simulink model "DC_DC_converter_closed_loop"  (R2019a)
settings: Solver=ode23tb  StartTime=0.0  StopTime=0.28  MaxStep=1e-7  RelTol=1e-7
values from neighbouring files (symbols this model uses):
  C = 33e-6    (= 3.3e-05)    [parameters_for_boost_converter_closed_loop.m]    (also in parameters_for_buck_converter_closed_loop.m)
  D = 1-((Vg+sqrt(Vg^2-4*V^2*((RL+Rdson)/R)))/(2*V))    [parameters_for_boost_converter_closed_loop.m]    (also in parameters_for_buck_converter_closed_loop.m = 0.425529411765)
  fsw = 100e3    (= 100000)    [parameters_for_boost_converter_closed_loop.m]    (also in parameters_for_buck_converter_closed_loop.m)
  H = 0.0075    [parameters_for_boost_converter_closed_loop.m]    (also in parameters_for_buck_converter_closed_loop.m)
  I = V/(R*(1-D))    [parameters_for_boost_converter_closed_loop.m]    (also in parameters_for_buck_converter_closed_loop.m = 11.7647058824)
  Kic_boost = 13590    [parameters_for_boost_converter_closed_loop.m]
  Kic_buck = 13529    [parameters_for_buck_converter_closed_loop.m]
  Kiv_boost = 25396    [parameters_for_boost_converter_closed_loop.m]
  Kiv_buck = 25428    [parameters_for_buck_converter_closed_loop.m]
  Kpc_boost = 0.618    [parameters_for_boost_converter_closed_loop.m]
  Kpc_buck = 0.6    [parameters_for_buck_converter_closed_loop.m]
  Kpv_boost = 15.62    [parameters_for_boost_converter_closed_loop.m]
  Kpv_buck = 6.53    [parameters_for_buck_converter_closed_loop.m]
  L = 250e-6    (= 0.00025)    [parameters_for_boost_converter_closed_loop.m]    (also in parameters_for_buck_converter_closed_loop.m)
  R = V/Iload    (= 80)    [parameters_for_boost_converter_closed_loop.m]    (also in parameters_for_buck_converter_closed_loop.m = 14.45)
  Resr = 6e-3    (= 0.006)    [parameters_for_boost_converter_closed_loop.m]    (also in parameters_for_buck_converter_closed_loop.m)
  Rf = 0.25    [parameters_for_boost_converter_closed_loop.m]    (also in parameters_for_buck_converter_closed_loop.m)
  RL = 10e-3    (= 0.01)    [parameters_for_boost_converter_closed_loop.m]    (also in parameters_for_buck_converter_closed_loop.m)
  Tsamp_dc = Tsw/2    (= 5e-06)    [parameters_for_boost_converter_closed_loop.m]    (also in parameters_for_buck_converter_closed_loop.m)
  V = 400    [parameters_for_boost_converter_closed_loop.m]    (also in parameters_for_buck_converter_closed_loop.m = 170)
  Vg = 170    [parameters_for_boost_converter_closed_loop.m]    (also in parameters_for_buck_converter_closed_loop.m = 400)
  VM = 4    [parameters_for_boost_converter_closed_loop.m]    (also in parameters_for_buck_converter_closed_loop.m)
  Vref = H*V    (= 3)    [parameters_for_boost_converter_closed_loop.m]    (also in parameters_for_buck_converter_closed_loop.m = 1.275)
libraries: powerlib x40, simulink x5
settings Model: Creator=Görkem  LastModifiedBy=gsahi
settings SolverCC: ZeroCrossAlgorithm=Adaptive
settings DebuggingCC: IgnoredZcDiagnostic=none

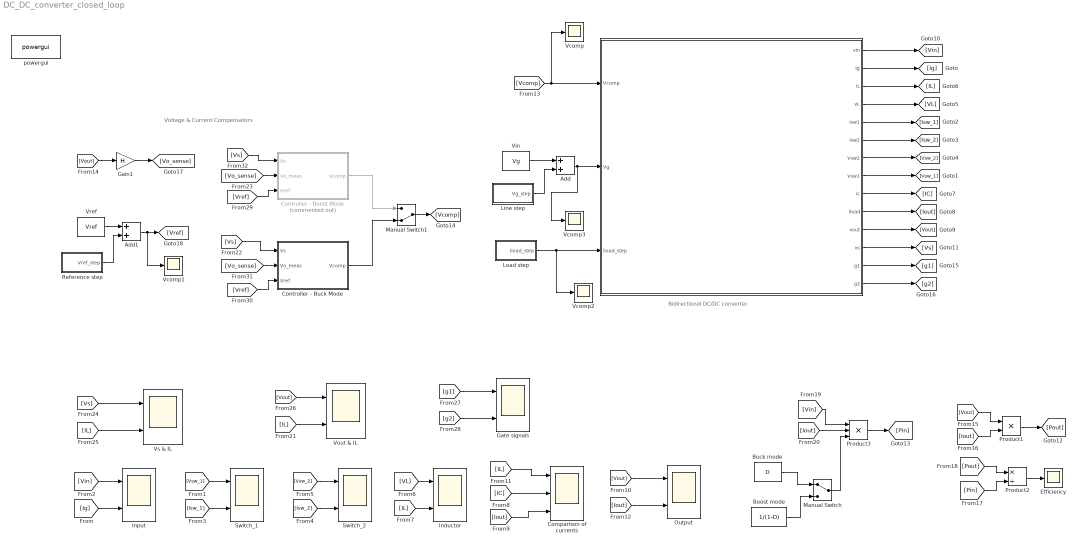
== system DC_DC_converter_closed_loop ==
  note: Voltage & Current Compensators
  note: Bidirectional DC/DC converter
  "   " : Subsystem
  Add : Sum
  Add1 : Sum
  Boost mode : Constant  Value=1/(1-D)
  Buck mode : Constant  Value=D
  Comparison of currents : Scope  NumInputPorts=3
  Controller - Boost Mode : Subsystem  Commented=on
  Controller - Buck Mode : Subsystem
  Efficiency : Scope
  Gain1 : Gain  Gain=H
  Gate signals : Scope  NumInputPorts=2
  Inductor : Scope  NumInputPorts=2
  Input : Scope  NumInputPorts=2
  Line step : Subsystem
  Load step : Subsystem
  Manual Switch : ManualSwitch
  Manual Switch1 : ManualSwitch  CurrentSetting=0
  "Output " : Scope  NumInputPorts=2
  Product1 : Product
  Product2 : Product  Inputs=*/
  Product3 : Product  Inputs=3
  Reference step : Subsystem
  Switch_1 : Scope  NumInputPorts=2
  Switch_2 : Scope  NumInputPorts=2
  Vcomp{,1..3} (4 alike) : Scope
  Vin : Constant  Value=Vg
  Vout & IL : Scope  NumInputPorts=2
  Vref : Constant  Value=Vref
  Vs & IL : Scope  NumInputPorts=2
  powergui : powerlib/powergui  Priority=1  SimulationMode=Continuous  SampleTime=5e-6  frequency=60  Iterations=50  frequencyindice=0  Pbase=100e6  ErrMax=1e-4  UnitsV=kV  UnitsW=MW  buscounter=0  FunctionMessages=off  echomessages=off  EnableUseOfTLC=off  CurrentSourceSwitches=off  DisableSnubberDevices=off  DisableRonSwitches=off  DisableVfSwitches=off  DisplayEquations=off  AutomaticDiscreteSolvers=off  SolverType=Tustin/Backward Euler (TBE)  Interpol=off  ExternalGateDelay=off  methode=off  Ts=100  x0status=blocks  SPID=on  SwTol=0  HookPort=off  NonlinearTolerance=0  nMaxIteration=15  ContinueOnMaxIteration=off  RestoreLinks=warning  ResistiveCurrentMeasurement=off  Frange=[0:2:500]  Ylog=off  Xlog=on  ShowGrid=off  save=off  variable=ZData  structure=0  ZoomFFT=off  StartTime=0.0  cycles=1  DisplayStyle=1  fundamental=60  FreqAxis=off  MaxFrequency=1000  frequencyindicesteady=1  RmsSteady=1  display=off
      settings: SourceProductName=Simscape Electrical
  wires:
  [Vin] -> Product3/1
  [Iout] -> Product3/2
  "   "/4(vL) -> [VL]
  "   "/6(isw2) -> [Isw_2]
  Product1/1 -> [Pout]
  "   "/9(ic) -> [IC]
  "   "/2(Ig) -> [Ig]
  "   "/11(vout) -> [Vout]
  Product3/1 -> [Pin]
  "   "/5(isw1) -> [Isw_1]
  [Vin] -> Input/1
  "   "/8(Vsw1) -> [Vsw_1]
  "   "/7(Vsw2) -> [Vsw_2]
  "   "/10(iload) -> [Iout]
  "   "/3(iL) -> [IL]
  [Iout] -> Comparison of currents/3
  [Pin] -> Product2/2
  [IL] -> Vout & IL/2
  [Pout] -> Product2/1
  "   "/1(vin) -> [Vin]
  Product2/1 -> Efficiency/1
  [Vout] -> Vout & IL/1
  [Isw_2] -> Switch_2/2
  [Iout] -> Product1/2
  [Vout] -> "Output "/1
  [IL] -> Inductor/2
  [VL] -> Inductor/1
  [Iout] -> "Output "/2
  [IC] -> Comparison of currents/2
  [Isw_1] -> Switch_1/2
  [Ig] -> Input/2
  [IL] -> Comparison of currents/1
  [Vsw_2] -> Switch_2/1
  [Vsw_1] -> Switch_1/1
  [Vout] -> Product1/1
  Buck mode/1 -> Manual Switch/1
  Boost mode/1 -> Manual Switch/2
  Manual Switch/1 -> Product3/3
  "   "/12(vs) -> [Vs]
  [Vout] -> Gain1/1
  [Vs] -> Vs & IL/1
  [IL] -> Vs & IL/2
  "   "/13(g1) -> [g1]
  "   "/14(g2) -> [g2]
  [g2] -> Gate signals/2
  [g1] -> Gate signals/1
  [Vcomp] -> Vcomp/1, "   "/1(Vcomp)
  Controller - Boost Mode/1("Vcomp ") -> Manual Switch1/1
  Controller - Buck Mode/1("Vcomp ") -> Manual Switch1/2
  Manual Switch1/1 -> [Vcomp]
  Gain1/1 -> [Vo_sense]
  [Vs] -> Controller - Buck Mode/1(Vs)
  [Vo_sense] -> Controller - Boost Mode/2(Vo_meas)
  [Vref] -> Controller - Boost Mode/3(Vref)
  [Vref] -> Controller - Buck Mode/3(Vref)
  [Vo_sense] -> Controller - Buck Mode/2(Vo_meas)
  [Vs] -> Controller - Boost Mode/1(Vs)
  Vin/1 -> Add/1
  Add/1 -> Vcomp3/1, "   "/2(Vg)
  Line step/1(Vg_step) -> Add/2
  Vref/1 -> Add1/1
  Reference step/1(Vref_step) -> Add1/2
  Add1/1 -> Vcomp1/1, [Vref]
  Load step/1(Iload_step) -> Vcomp2/1, "   "/3(iload_step)

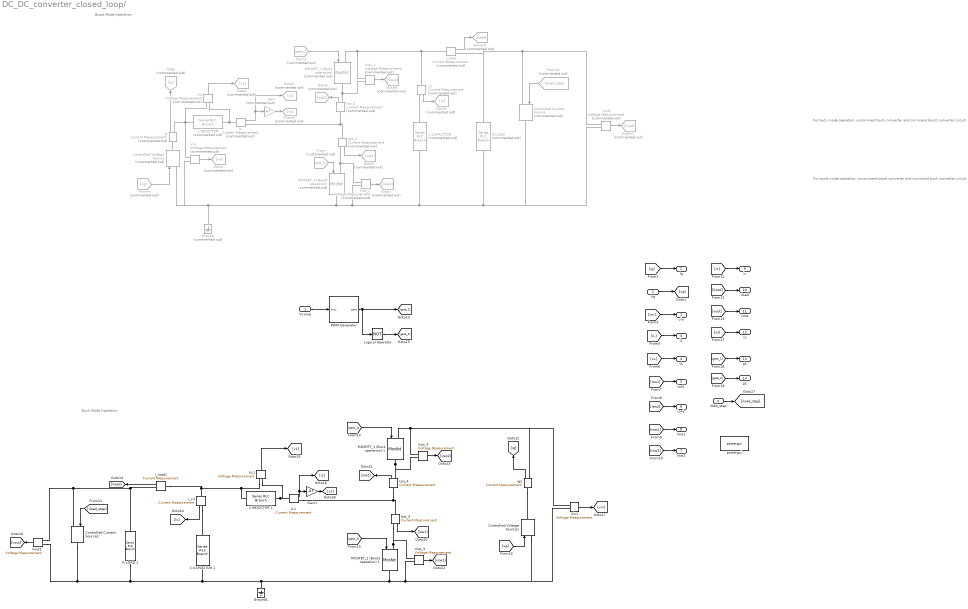
== system DC_DC_converter_closed_loop/    ==
  note: For buck mode operation, uncomment buck converter and command boost converter circuit
  note: Buck Mode Operation
  note: Boost Mode Operation
  note: For boost mode operation, uncomment boost converter and command buck converter circuit
  Vcomp : Inport
  Vg : Inport  Port=2
  iload_step : Inport  Port=3
  "C:CAPACITOR " : powerlib/Elements/Series RLC Branch  Commented=on  LConnTagsString=__new0  RConnTagsString=__new0  BranchType=RC  Resistance=Resr  Inductance=1e-3  SetiL0=off  InitialCurrent=0  Capacitance=C  Setx0=off  InitialVoltage=0  Measurements=None
      settings: SourceProductName=Simscape Electrical
  C:CAPACITOR 1 : powerlib/Elements/Series RLC Branch  LConnTagsString=__new0  RConnTagsString=__new0  BranchType=RC  Resistance=Resr  Inductance=1e-3  SetiL0=off  InitialCurrent=0  Capacitance=C  Setx0=off  InitialVoltage=0  Measurements=None
      settings: SourceProductName=Simscape Electrical
  Controlled Current Source : powerlib/Electrical Sources/Controlled Current Source  Commented=on  Initialize=on  Source_Type=AC  Amplitude=0  Phase=0  Frequency=0  Measurements=None
      settings: SourceProductName=Simscape Electrical
  Controlled Current Source1 : powerlib/Electrical Sources/Controlled Current Source  Initialize=on  Source_Type=AC  Amplitude=0  Phase=0  Frequency=0  Measurements=None
      settings: SourceProductName=Simscape Electrical
  Controlled Voltage Source : powerlib/Electrical Sources/Controlled Voltage Source  Commented=on  Initialize=on  Source_Type=DC  Amplitude=0  Phase=0  Frequency=0  Measurements=None
      settings: SourceProductName=Simscape Electrical
  Controlled Voltage Source1 : powerlib/Electrical Sources/Controlled Voltage Source  Initialize=on  Source_Type=DC  Amplitude=0  Phase=0  Frequency=0  Measurements=None
      settings: SourceProductName=Simscape Electrical
  From : From  Commented=on  GotoTag=gate_1
  From1 : From  Commented=on  GotoTag=gate_2
  From20 : From  Commented=on  GotoTag=iload_step
  From4 : From  Commented=on  GotoTag=vg
  Gain : Gain  Commented=on  Gain=Rf
  Gain1 : Gain  Gain=-Rf
  Goto : Goto  Commented=on  GotoTag=ig
  Goto10 : Goto  Commented=on  GotoTag=iload
  Goto11 : Goto  Commented=on  GotoTag=vout
  Goto2 : Goto  Commented=on  GotoTag=vin
  Goto25 : Goto  Commented=on  GotoTag=vs
  Goto3 : Goto  Commented=on  GotoTag=iL
  Goto4 : Goto  Commented=on  GotoTag=vL
  Goto5 : Goto  Commented=on  GotoTag=isw1
  Goto6 : Goto  Commented=on  GotoTag=isw2
  Goto7 : Goto  Commented=on  GotoTag=vsw1
  Goto8 : Goto  Commented=on  GotoTag=vsw2
  Goto9 : Goto  Commented=on  GotoTag=ic
  Ground : powerlib/Elements/Ground  Commented=on  LConnTagsString=a
      settings: SourceProductName=Simscape Electrical
  Ground1 : powerlib/Elements/Ground  LConnTagsString=a
      settings: SourceProductName=Simscape Electrical
  IL : powerlib/Measurements/Current Measurement  Commented=on  PhasorSimulation=off  OutputType=Complex  PSBequivalent=0
      settings: SourceProductName=Simscape Electrical
  IL1 : powerlib/Measurements/Current Measurement  PhasorSimulation=off  OutputType=Complex  PSBequivalent=0
      settings: SourceProductName=Simscape Electrical
  Isw_1 : powerlib/Measurements/Current Measurement  Commented=on  PhasorSimulation=off  OutputType=Complex  PSBequivalent=0
      settings: SourceProductName=Simscape Electrical
  Isw_2 : powerlib/Measurements/Current Measurement  Commented=on  PhasorSimulation=off  OutputType=Complex  PSBequivalent=0
      settings: SourceProductName=Simscape Electrical
  Isw_3 : powerlib/Measurements/Current Measurement  PhasorSimulation=off  OutputType=Complex  PSBequivalent=0
      settings: SourceProductName=Simscape Electrical
  Isw_4 : powerlib/Measurements/Current Measurement  PhasorSimulation=off  OutputType=Complex  PSBequivalent=0
      settings: SourceProductName=Simscape Electrical
  "L:INDUCTOR " : powerlib/Elements/Series RLC Branch  Commented=on  LConnTagsString=__new0  RConnTagsString=__new0  BranchType=RL  Resistance=RL  Inductance=L  SetiL0=off  InitialCurrent=0  Capacitance=1e-6  Setx0=off  InitialVoltage=0  Measurements=None
      settings: SourceProductName=Simscape Electrical
  L:INDUCTOR 1 : powerlib/Elements/Series RLC Branch  LConnTagsString=__new0  RConnTagsString=__new0  BranchType=RL  Resistance=RL  Inductance=L  SetiL0=off  InitialCurrent=0  Capacitance=1e-6  Setx0=off  InitialVoltage=0  Measurements=None
      settings: SourceProductName=Simscape Electrical
  Logical Operator : Logic  Operator=NOT  AllPortsSameDT=off  OutDataTypeStr=boolean
  "MOSFET_1 (Buck operation) " : powerlib/Power Electronics/Mosfet  Commented=on  Ron=Rdson  Lon=0  Rd=0  Vfd=Vf  IC=0  Rs=1e5  Cs=inf  Measurements=off
      settings: SourceProductName=Simscape Electrical
  MOSFET_1 (Buck operation) 1 : powerlib/Power Electronics/Mosfet  Ron=Rdson  Lon=0  Rd=0  Vfd=Vf  IC=0  Rs=1e5  Cs=inf  Measurements=off
      settings: SourceProductName=Simscape Electrical
  "MOSFET_2 (Boost operation) " : powerlib/Power Electronics/Mosfet  Commented=on  Ron=Rdson  Lon=0  Rd=0  Vfd=Vf  IC=0  Rs=1e5  Cs=inf  Measurements=off
      settings: SourceProductName=Simscape Electrical
  MOSFET_2 (Boost operation) 1 : powerlib/Power Electronics/Mosfet  Ron=Rdson  Lon=0  Rd=0  Vfd=Vf  IC=0  Rs=1e5  Cs=inf  Measurements=off
      settings: SourceProductName=Simscape Electrical
  PWM Generator : Subsystem
  "R:LOAD " : powerlib/Elements/Series RLC Branch  Commented=on  LConnTagsString=__new0  RConnTagsString=__new0  BranchType=R  Resistance=R  Inductance=1e-3  SetiL0=off  InitialCurrent=0  Capacitance=47e-6  Setx0=off  InitialVoltage=0  Measurements=None
      settings: SourceProductName=Simscape Electrical
  R:LOAD 1 : powerlib/Elements/Series RLC Branch  LConnTagsString=__new0  RConnTagsString=__new0  BranchType=R  Resistance=R  Inductance=1e-3  SetiL0=off  InitialCurrent=0  Capacitance=47e-6  Setx0=off  InitialVoltage=0  Measurements=None
      settings: SourceProductName=Simscape Electrical
  VL : powerlib/Measurements/Voltage Measurement  Commented=on  PhasorSimulation=off  OutputType=Complex  PSBequivalent=0
      settings: SourceProductName=Simscape Electrical
  VL1 : powerlib/Measurements/Voltage Measurement  PhasorSimulation=off  OutputType=Complex  PSBequivalent=0
      settings: SourceProductName=Simscape Electrical
  Vin : powerlib/Measurements/Voltage Measurement  Commented=on  PhasorSimulation=off  OutputType=Complex  PSBequivalent=0
      settings: SourceProductName=Simscape Electrical
  Vin1 : powerlib/Measurements/Voltage Measurement  PhasorSimulation=off  OutputType=Complex  PSBequivalent=0
      settings: SourceProductName=Simscape Electrical
  Vout : powerlib/Measurements/Voltage Measurement  Commented=on  PhasorSimulation=off  OutputType=Complex  PSBequivalent=0
      settings: SourceProductName=Simscape Electrical
  Vout1 : powerlib/Measurements/Voltage Measurement  PhasorSimulation=off  OutputType=Complex  PSBequivalent=0
      settings: SourceProductName=Simscape Electrical
  Vsw_1 : powerlib/Measurements/Voltage Measurement  Commented=on  PhasorSimulation=off  OutputType=Complex  PSBequivalent=0
      settings: SourceProductName=Simscape Electrical
  Vsw_2 : powerlib/Measurements/Voltage Measurement  Commented=on  PhasorSimulation=off  OutputType=Complex  PSBequivalent=0
      settings: SourceProductName=Simscape Electrical
  Vsw_3 : powerlib/Measurements/Voltage Measurement  PhasorSimulation=off  OutputType=Complex  PSBequivalent=0
      settings: SourceProductName=Simscape Electrical
  Vsw_4 : powerlib/Measurements/Voltage Measurement  PhasorSimulation=off  OutputType=Complex  PSBequivalent=0
      settings: SourceProductName=Simscape Electrical
  i_c : powerlib/Measurements/Current Measurement  Commented=on  PhasorSimulation=off  OutputType=Complex  PSBequivalent=0
      settings: SourceProductName=Simscape Electrical
  i_c1 : powerlib/Measurements/Current Measurement  PhasorSimulation=off  OutputType=Complex  PSBequivalent=0
      settings: SourceProductName=Simscape Electrical
  i_load : powerlib/Measurements/Current Measurement  Commented=on  PhasorSimulation=off  OutputType=Complex  PSBequivalent=0
      settings: SourceProductName=Simscape Electrical
  i_load1 : powerlib/Measurements/Current Measurement  PhasorSimulation=off  OutputType=Complex  PSBequivalent=0
      settings: SourceProductName=Simscape Electrical
  ig : powerlib/Measurements/Current Measurement  Commented=on  PhasorSimulation=off  OutputType=Complex  PSBequivalent=0
      settings: SourceProductName=Simscape Electrical
  ig1 : powerlib/Measurements/Current Measurement  PhasorSimulation=off  OutputType=Complex  PSBequivalent=0
      settings: SourceProductName=Simscape Electrical
  powergui : powerlib/powergui  Priority=1  SimulationMode=Continuous  SampleTime=50e-6  frequency=60  Iterations=50  frequencyindice=0  Pbase=100e6  ErrMax=1e-4  UnitsV=kV  UnitsW=MW  buscounter=0  FunctionMessages=off  echomessages=off  EnableUseOfTLC=off  CurrentSourceSwitches=off  DisableSnubberDevices=off  DisableRonSwitches=off  DisableVfSwitches=off  DisplayEquations=off  AutomaticDiscreteSolvers=off  SolverType=Tustin/Backward Euler (TBE)  Interpol=off  ExternalGateDelay=off  methode=off  Ts=100  x0status=blocks  SPID=on  SwTol=0  HookPort=off  NonlinearTolerance=0  nMaxIteration=15  ContinueOnMaxIteration=off  RestoreLinks=warning  ResistiveCurrentMeasurement=off  Frange=[0:2:500]  Ylog=off  Xlog=on  ShowGrid=off  save=off  variable=ZData  structure=0  ZoomFFT=off  StartTime=0.0  cycles=1  DisplayStyle=1  fundamental=60  FreqAxis=off  MaxFrequency=1000  frequencyindicesteady=1  RmsSteady=1  display=off
      settings: SourceProductName=Simscape Electrical
  vin : Outport
  Ig : Outport  Port=2
  iL : Outport  Port=3
  vL : Outport  Port=4
  isw1 : Outport  Port=5
  isw2 : Outport  Port=6
  Vsw2 : Outport  Port=7
  Vsw1 : Outport  Port=8
  ic : Outport  Port=9
  iload : Outport  Port=10
  vout : Outport  Port=11
  vs : Outport  Port=12
  g1 : Outport  Port=13
  g2 : Outport  Port=14
  wires:
  PWM Generator/1(gate) -> Logical Operator/1, [gate_1]
  Logical Operator/1 -> [gate_2]
  Vcomp/1 -> PWM Generator/1(duty)
  From/1 -> "MOSFET_2 (Boost operation) "/1
  From1/1 -> "MOSFET_1 (Buck operation) "/1
  Vout/1 -> Goto11/1
  IL/1 -> Gain/1, Goto3/1
  VL/1 -> Goto4/1
  ig/1 -> Goto/1
  Isw_1/1 -> Goto5/1
  Isw_2/1 -> Goto6/1
  Vsw_1/1 -> Goto7/1
  Vsw_2/1 -> Goto8/1
  i_c/1 -> Goto9/1
  [ig] -> Ig/1
  Vg/1 -> [vg]
  From4/1 -> Controlled Voltage Source/1
  Vin/1 -> Goto2/1
  [vin] -> vin/1
  [iL] -> iL/1
  [vL] -> vL/1
  [isw1] -> isw1/1
  [isw2] -> isw2/1
  [vsw1] -> Vsw1/1
  [vsw2] -> Vsw2/1
  [ic] -> ic/1
  [iload] -> iload/1
  [vout] -> vout/1
  [gate_1] -> MOSFET_1 (Buck operation) 1/1
  Vsw_4/1 -> [vsw2]
  [gate_2] -> MOSFET_2 (Boost operation) 1/1
  VL1/1 -> [vL]
  Vsw_3/1 -> [vsw1]
  Isw_3/1 -> [isw1]
  IL1/1 -> [iL], Gain1/1
  Isw_4/1 -> [isw2]
  [vg] -> Controlled Voltage Source1/1
  ig1/1 -> [ig]
  Vin1/1 -> [vin]
  Vout1/1 -> [vout]
  i_c1/1 -> [ic]
  [vs] -> vs/1
  [gate_2] -> g2/1
  [gate_1] -> g1/1
  Gain/1 -> Goto25/1
  Gain1/1 -> [vs]
  From20/1 -> Controlled Current Source/1
  iload_step/1 -> [iload_step]
  i_load/1 -> Goto10/1
  [iload_step] -> Controlled Current Source1/1
  i_load1/1 -> [iload]
  connections:
  Vout/LConn1 -- i_load/RConn1 -- "R:LOAD "/LConn1 -- Controlled Current Source/LConn1
  "C:CAPACITOR "/RConn1 -- Controlled Current Source/RConn1 -- Vout/LConn2 -- "R:LOAD "/RConn1 -- Vsw_1/LConn2 -- Vin/LConn2 -- Controlled Voltage Source/LConn1 -- Ground/LConn1 -- "MOSFET_2 (Boost operation) "/RConn1
  Isw_1/LConn1 -- IL/RConn1 -- Isw_2/LConn1
  VL/LConn1 -- Vin/LConn1 -- "L:INDUCTOR "/LConn1 -- ig/RConn1
  IL/LConn1 -- VL/LConn2 -- "L:INDUCTOR "/RConn1
  ig/LConn1 -- Controlled Voltage Source/RConn1
  Isw_1/RConn1 -- Vsw_1/LConn1 -- "MOSFET_2 (Boost operation) "/LConn1
  Isw_2/RConn1 -- Vsw_2/LConn1 -- "MOSFET_1 (Buck operation) "/RConn1
  i_c/RConn1 -- "C:CAPACITOR "/LConn1
  MOSFET_1 (Buck operation) 1/RConn1 -- Isw_4/RConn1 -- Vsw_4/LConn1
  MOSFET_2 (Boost operation) 1/LConn1 -- Isw_3/RConn1 -- Vsw_3/LConn1
  Vout1/LConn2 -- Ground1/LConn1 -- Vin1/LConn2 -- Controlled Voltage Source1/LConn1 -- Vsw_3/LConn2 -- MOSFET_2 (Boost operation) 1/RConn1 -- C:CAPACITOR 1/RConn1 -- R:LOAD 1/RConn1 -- Controlled Current Source1/RConn1
  Isw_4/LConn1 -- Isw_3/LConn1 -- IL1/RConn1
  L:INDUCTOR 1/RConn1 -- IL1/LConn1 -- VL1/LConn2
  Vout1/LConn1 -- Controlled Current Source1/LConn1 -- i_load1/RConn1 -- R:LOAD 1/LConn1
  i_c1/RConn1 -- C:CAPACITOR 1/LConn1
  Vsw_4/LConn2 -- Vin1/LConn1 -- ig1/RConn1 -- MOSFET_1 (Buck operation) 1/LConn1
  ig1/LConn1 -- Controlled Voltage Source1/RConn1
  i_c/LConn1 -- i_load/LConn1 -- Vsw_2/LConn2 -- "MOSFET_1 (Buck operation) "/LConn1
  L:INDUCTOR 1/LConn1 -- i_load1/LConn1 -- i_c1/LConn1 -- VL1/LConn1

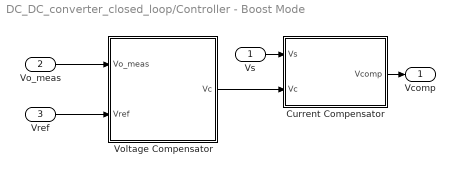
== system DC_DC_converter_closed_loop/Controller - Boost Mode ==
  Vs : Inport
  Vo_meas : Inport  Port=2
  Vref : Inport  Port=3
  Current Compensator : Subsystem
  "Voltage Compensator " : Subsystem
  "Vcomp " : Outport
  wires:
  Vs/1 -> Current Compensator/1(Vs)
  "Voltage Compensator "/1(Vc) -> Current Compensator/2(Vc)
  Vref/1 -> "Voltage Compensator "/2(Vref)
  Current Compensator/1(Vcomp) -> "Vcomp "/1
  Vo_meas/1 -> "Voltage Compensator "/1("Vo_meas ")

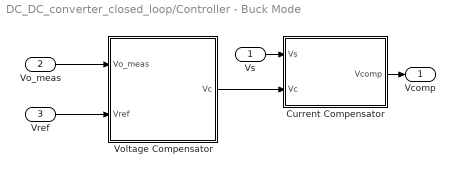
== system DC_DC_converter_closed_loop/Controller - Buck Mode ==
  Vs : Inport
  Vo_meas : Inport  Port=2
  Vref : Inport  Port=3
  Current Compensator : Subsystem
  "Voltage Compensator " : Subsystem
  "Vcomp " : Outport
  wires:
  Vs/1 -> Current Compensator/1(Vs)
  "Voltage Compensator "/1(Vc) -> Current Compensator/2(Vc)
  Vref/1 -> "Voltage Compensator "/2(Vref)
  Current Compensator/1(Vcomp) -> "Vcomp "/1
  Vo_meas/1 -> "Voltage Compensator "/1("Vo_meas ")

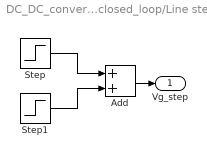
== system DC_DC_converter_closed_loop/Line step ==
  Add : Sum
  Step : Step  Time=0.12  After=10  SampleTime=0
  Step1 : Step  Time=0.16  After=-10  SampleTime=0
  Vg_step : Outport
  wires:
  Add/1 -> Vg_step/1
  Step/1 -> Add/1
  Step1/1 -> Add/2

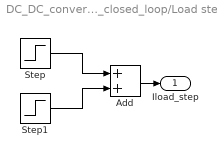
== system DC_DC_converter_closed_loop/Load step ==
  Add : Sum
  Step : Step  Time=0.20  After=V/R  SampleTime=0
  Step1 : Step  Time=0.24  After=-V/R  SampleTime=0
  Iload_step : Outport
  wires:
  Add/1 -> Iload_step/1
  Step/1 -> Add/1
  Step1/1 -> Add/2

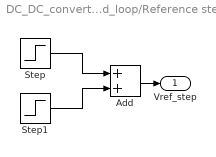
== system DC_DC_converter_closed_loop/Reference step ==
  Add : Sum
  Step : Step  Time=0.04  After=H*V*0.5  SampleTime=0
  Step1 : Step  Time=0.08  After=-H*V*0.5  SampleTime=0
  Vref_step : Outport
  wires:
  Add/1 -> Vref_step/1
  Step/1 -> Add/1
  Step1/1 -> Add/2

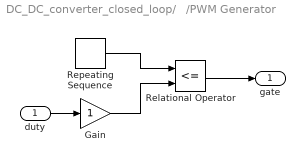
== system DC_DC_converter_closed_loop/   /PWM Generator ==
  duty : Inport
  Gain : Gain
  Relational Operator : RelationalOperator  Operator=<=  OutDataTypeStr=boolean  RndMeth=Simplest
  Repeating Sequence : simulink/Sources/Repeating Sequence  rep_seq_t=[0 0.5/fsw 1/fsw]  rep_seq_y=[0 VM 0]
  gate : Outport
  wires:
  Repeating Sequence/1 -> Relational Operator/1
  Relational Operator/1 -> gate/1
  duty/1 -> Gain/1
  Gain/1 -> Relational Operator/2

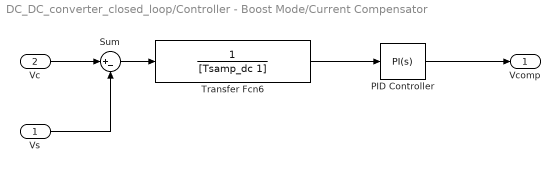
== system DC_DC_converter_closed_loop/Controller - Boost Mode/Current Compensator ==
  Vs : Inport
  Vc : Inport  Port=2
  PID Controller : simulink/Continuous/PID Controller  Controller=PI  Form=Parallel  TimeDomain=Continuous-time  SampleTime=-1  IntegratorMethod=Forward Euler  FilterMethod=Forward Euler  ControllerParametersSource=internal  P=Kpc_boost  I=Kic_boost  D=0  UseFilter=on  N=100  TunerSelectOption=Transfer Function Based (PID Tuner App)  InitialConditionSource=internal  InitialConditionForIntegrator=0  InitialConditionForFilter=0  DifferentiatorICPrevScaledInput=0  ExternalReset=none  TrackingMode=off  Kt=1  LimitOutput=off  UpperSaturationLimit=VM  LowerSaturationLimit=-VM  LinearizeAsGain=on  AntiWindupMode=none  Kb=1  POutMin=[]  POutMax=[]  IOutMin=[]  IOutMax=[]  DOutMin=[]  DOutMax=[]  NOutMin=[]  NOutMax=[]  SumOutMin=[]  SumOutMax=[]  SaturationOutMin=[]  SaturationOutMax=[]  PParamMin=[]  PParamMax=[]  IParamMin=[]  IParamMax=[]  DParamMin=[]  DParamMax=[]  NParamMin=[]  NParamMax=[]  KbParamMin=[]  KbParamMax=[]  KtParamMin=[]  KtParamMax=[]  KbOutMin=[]  KbOutMax=[]  KtOutMin=[]  KtOutMax=[]  IntegratorOutMin=[]  IntegratorOutMax=[]  FilterOutMin=[]  FilterOutMax=[]  SumI1OutMin=[]  SumI1OutMax=[]  SumI2OutMin=[]  SumI2OutMax=[]  SumI3OutMin=[]  SumI3OutMax=[]  SumI4OutMin=[]  SumI4OutMax=[]  SumDOutMin=[]  SumDOutMax=[]  DifferentiatorOutMin=[]  DifferentiatorOutMax=[]  FilterDiffOutCoefMin=[]  FilterDiffOutCoefMax=[]  ReciprocalOutMin=[]  ReciprocalOutMax=[]  SumDenOutMin=[]  SumDenOutMax=[]  SumNumOutMin=[]  SumNumOutMax=[]  DivideOutMin=[]  DivideOutMax=[]  IntegratorContinuousStateAttributes=''  IntegratorStateMustResolveToSignalObject=off  IntegratorRTWStateStorageClass=Auto  FilterContinuousStateAttributes=''  FilterStateMustResolveToSignalObject=off  FilterRTWStateStorageClass=Auto  ParallelPVariant=InternalParameters  IdealPVariant=Disabled  IVariant=InternalParameters  DVariant=Disabled  IntegratorVariant=Continuous  SatVariant=Disabled  AWVariant=Passthrough  PCopyVariant=Disabled  TRVariant=Disabled  FdbkBlocksVariant=Forward  IdealPFdbkVariant=Disabled  SatFdbkVariant=Disabled  DerivativeFilterVariant=Disabled  NVariant=Disabled  NCopyVariant=Disabled_SignalSpec  FilterICVariant=Disabled  IntegratorICVariant=InternalICs  ExternalResetVariant=Disabled  TRSumVariant=Passthrough  SumFdbkVariant=Disabled  SumVariant=Sum_PI
  Sum : Sum  Inputs=|+-
  Transfer Fcn6 : TransferFcn  Denominator=[Tsamp_dc 1]
  Vcomp : Outport
  wires:
  Vc/1 -> Sum/1
  Vs/1 -> Sum/2
  Sum/1 -> Transfer Fcn6/1
  Transfer Fcn6/1 -> PID Controller/1
  PID Controller/1 -> Vcomp/1

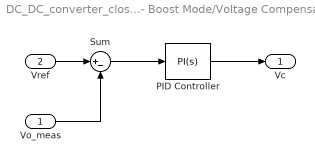
== system DC_DC_converter_closed_loop/Controller - Boost Mode/Voltage Compensator  ==
  "Vo_meas " : Inport
  Vref : Inport  Port=2
  PID Controller : simulink/Continuous/PID Controller  Controller=PI  Form=Parallel  TimeDomain=Continuous-time  SampleTime=-1  IntegratorMethod=Forward Euler  FilterMethod=Forward Euler  ControllerParametersSource=internal  P=Kpv_boost  I=Kiv_boost  D=0  UseFilter=on  N=100  TunerSelectOption=Transfer Function Based (PID Tuner App)  InitialConditionSource=internal  InitialConditionForIntegrator=0  InitialConditionForFilter=0  DifferentiatorICPrevScaledInput=0  ExternalReset=none  TrackingMode=off  Kt=1  LimitOutput=on  UpperSaturationLimit=2.5*Rf*I  LowerSaturationLimit=-2.5*Rf*I  LinearizeAsGain=on  AntiWindupMode=none  Kb=1  POutMin=[]  POutMax=[]  IOutMin=[]  IOutMax=[]  DOutMin=[]  DOutMax=[]  NOutMin=[]  NOutMax=[]  SumOutMin=[]  SumOutMax=[]  SaturationOutMin=[]  SaturationOutMax=[]  PParamMin=[]  PParamMax=[]  IParamMin=[]  IParamMax=[]  DParamMin=[]  DParamMax=[]  NParamMin=[]  NParamMax=[]  KbParamMin=[]  KbParamMax=[]  KtParamMin=[]  KtParamMax=[]  KbOutMin=[]  KbOutMax=[]  KtOutMin=[]  KtOutMax=[]  IntegratorOutMin=[]  IntegratorOutMax=[]  FilterOutMin=[]  FilterOutMax=[]  SumI1OutMin=[]  SumI1OutMax=[]  SumI2OutMin=[]  SumI2OutMax=[]  SumI3OutMin=[]  SumI3OutMax=[]  SumI4OutMin=[]  SumI4OutMax=[]  SumDOutMin=[]  SumDOutMax=[]  DifferentiatorOutMin=[]  DifferentiatorOutMax=[]  FilterDiffOutCoefMin=[]  FilterDiffOutCoefMax=[]  ReciprocalOutMin=[]  ReciprocalOutMax=[]  SumDenOutMin=[]  SumDenOutMax=[]  SumNumOutMin=[]  SumNumOutMax=[]  DivideOutMin=[]  DivideOutMax=[]  IntegratorContinuousStateAttributes=''  IntegratorStateMustResolveToSignalObject=off  IntegratorRTWStateStorageClass=Auto  FilterContinuousStateAttributes=''  FilterStateMustResolveToSignalObject=off  FilterRTWStateStorageClass=Auto  ParallelPVariant=InternalParameters  IdealPVariant=Disabled  IVariant=InternalParameters  DVariant=Disabled  IntegratorVariant=Continuous  SatVariant=Enabled  AWVariant=Passthrough  PCopyVariant=Disabled  TRVariant=Disabled  FdbkBlocksVariant=Forward  IdealPFdbkVariant=Disabled  SatFdbkVariant=Disabled  DerivativeFilterVariant=Disabled  NVariant=Disabled  NCopyVariant=Disabled_SignalSpec  FilterICVariant=Disabled  IntegratorICVariant=InternalICs  ExternalResetVariant=Disabled  TRSumVariant=Passthrough  SumFdbkVariant=Disabled  SumVariant=Sum_PI
  Sum : Sum  Inputs=|+-
  Vc : Outport
  wires:
  "Vo_meas "/1 -> Sum/2
  Vref/1 -> Sum/1
  Sum/1 -> PID Controller/1
  PID Controller/1 -> Vc/1

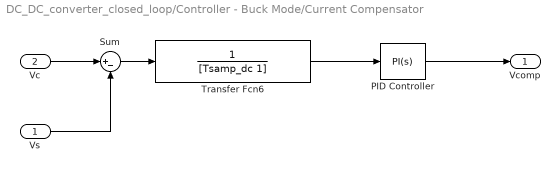
== system DC_DC_converter_closed_loop/Controller - Buck Mode/Current Compensator ==
  Vs : Inport
  Vc : Inport  Port=2
  PID Controller : simulink/Continuous/PID Controller  Controller=PI  Form=Parallel  TimeDomain=Continuous-time  SampleTime=-1  IntegratorMethod=Forward Euler  FilterMethod=Forward Euler  ControllerParametersSource=internal  P=Kpc_buck  I=Kic_buck  D=0  UseFilter=on  N=100  TunerSelectOption=Transfer Function Based (PID Tuner App)  InitialConditionSource=internal  InitialConditionForIntegrator=0  InitialConditionForFilter=0  DifferentiatorICPrevScaledInput=0  ExternalReset=none  TrackingMode=off  Kt=1  LimitOutput=off  UpperSaturationLimit=VM  LowerSaturationLimit=0  LinearizeAsGain=on  AntiWindupMode=none  Kb=1  POutMin=[]  POutMax=[]  IOutMin=[]  IOutMax=[]  DOutMin=[]  DOutMax=[]  NOutMin=[]  NOutMax=[]  SumOutMin=[]  SumOutMax=[]  SaturationOutMin=[]  SaturationOutMax=[]  PParamMin=[]  PParamMax=[]  IParamMin=[]  IParamMax=[]  DParamMin=[]  DParamMax=[]  NParamMin=[]  NParamMax=[]  KbParamMin=[]  KbParamMax=[]  KtParamMin=[]  KtParamMax=[]  KbOutMin=[]  KbOutMax=[]  KtOutMin=[]  KtOutMax=[]  IntegratorOutMin=[]  IntegratorOutMax=[]  FilterOutMin=[]  FilterOutMax=[]  SumI1OutMin=[]  SumI1OutMax=[]  SumI2OutMin=[]  SumI2OutMax=[]  SumI3OutMin=[]  SumI3OutMax=[]  SumI4OutMin=[]  SumI4OutMax=[]  SumDOutMin=[]  SumDOutMax=[]  DifferentiatorOutMin=[]  DifferentiatorOutMax=[]  FilterDiffOutCoefMin=[]  FilterDiffOutCoefMax=[]  ReciprocalOutMin=[]  ReciprocalOutMax=[]  SumDenOutMin=[]  SumDenOutMax=[]  SumNumOutMin=[]  SumNumOutMax=[]  DivideOutMin=[]  DivideOutMax=[]  IntegratorContinuousStateAttributes=''  IntegratorStateMustResolveToSignalObject=off  IntegratorRTWStateStorageClass=Auto  FilterContinuousStateAttributes=''  FilterStateMustResolveToSignalObject=off  FilterRTWStateStorageClass=Auto  ParallelPVariant=InternalParameters  IdealPVariant=Disabled  IVariant=InternalParameters  DVariant=Disabled  IntegratorVariant=Continuous  SatVariant=Disabled  AWVariant=Passthrough  PCopyVariant=Disabled  TRVariant=Disabled  FdbkBlocksVariant=Forward  IdealPFdbkVariant=Disabled  SatFdbkVariant=Disabled  DerivativeFilterVariant=Disabled  NVariant=Disabled  NCopyVariant=Disabled_SignalSpec  FilterICVariant=Disabled  IntegratorICVariant=InternalICs  ExternalResetVariant=Disabled  TRSumVariant=Passthrough  SumFdbkVariant=Disabled  SumVariant=Sum_PI
  Sum : Sum  Inputs=|+-
  Transfer Fcn6 : TransferFcn  Denominator=[Tsamp_dc 1]
  Vcomp : Outport
  wires:
  Vc/1 -> Sum/1
  Vs/1 -> Sum/2
  Sum/1 -> Transfer Fcn6/1
  Transfer Fcn6/1 -> PID Controller/1
  PID Controller/1 -> Vcomp/1

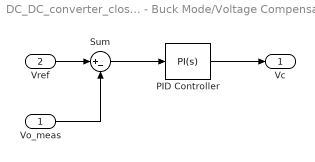
== system DC_DC_converter_closed_loop/Controller - Buck Mode/Voltage Compensator  ==
  "Vo_meas " : Inport
  Vref : Inport  Port=2
  PID Controller : simulink/Continuous/PID Controller  Controller=PI  Form=Parallel  TimeDomain=Continuous-time  SampleTime=-1  IntegratorMethod=Forward Euler  FilterMethod=Forward Euler  ControllerParametersSource=internal  P=Kpv_buck  I=Kiv_buck  D=0  UseFilter=on  N=100  TunerSelectOption=Transfer Function Based (PID Tuner App)  InitialConditionSource=internal  InitialConditionForIntegrator=0  InitialConditionForFilter=0  DifferentiatorICPrevScaledInput=0  ExternalReset=none  TrackingMode=off  Kt=1  LimitOutput=off  UpperSaturationLimit=Rf*I  LowerSaturationLimit=-inf  LinearizeAsGain=on  AntiWindupMode=none  Kb=1  POutMin=[]  POutMax=[]  IOutMin=[]  IOutMax=[]  DOutMin=[]  DOutMax=[]  NOutMin=[]  NOutMax=[]  SumOutMin=[]  SumOutMax=[]  SaturationOutMin=[]  SaturationOutMax=[]  PParamMin=[]  PParamMax=[]  IParamMin=[]  IParamMax=[]  DParamMin=[]  DParamMax=[]  NParamMin=[]  NParamMax=[]  KbParamMin=[]  KbParamMax=[]  KtParamMin=[]  KtParamMax=[]  KbOutMin=[]  KbOutMax=[]  KtOutMin=[]  KtOutMax=[]  IntegratorOutMin=[]  IntegratorOutMax=[]  FilterOutMin=[]  FilterOutMax=[]  SumI1OutMin=[]  SumI1OutMax=[]  SumI2OutMin=[]  SumI2OutMax=[]  SumI3OutMin=[]  SumI3OutMax=[]  SumI4OutMin=[]  SumI4OutMax=[]  SumDOutMin=[]  SumDOutMax=[]  DifferentiatorOutMin=[]  DifferentiatorOutMax=[]  FilterDiffOutCoefMin=[]  FilterDiffOutCoefMax=[]  ReciprocalOutMin=[]  ReciprocalOutMax=[]  SumDenOutMin=[]  SumDenOutMax=[]  SumNumOutMin=[]  SumNumOutMax=[]  DivideOutMin=[]  DivideOutMax=[]  IntegratorContinuousStateAttributes=''  IntegratorStateMustResolveToSignalObject=off  IntegratorRTWStateStorageClass=Auto  FilterContinuousStateAttributes=''  FilterStateMustResolveToSignalObject=off  FilterRTWStateStorageClass=Auto  ParallelPVariant=InternalParameters  IdealPVariant=Disabled  IVariant=InternalParameters  DVariant=Disabled  IntegratorVariant=Continuous  SatVariant=Disabled  AWVariant=Passthrough  PCopyVariant=Disabled  TRVariant=Disabled  FdbkBlocksVariant=Forward  IdealPFdbkVariant=Disabled  SatFdbkVariant=Disabled  DerivativeFilterVariant=Disabled  NVariant=Disabled  NCopyVariant=Disabled_SignalSpec  FilterICVariant=Disabled  IntegratorICVariant=InternalICs  ExternalResetVariant=Disabled  TRSumVariant=Passthrough  SumFdbkVariant=Disabled  SumVariant=Sum_PI
  Sum : Sum  Inputs=|+-
  Vc : Outport
  wires:
  "Vo_meas "/1 -> Sum/2
  Vref/1 -> Sum/1
  Sum/1 -> PID Controller/1
  PID Controller/1 -> Vc/1
